simulink model "robot_dynamics_model"  (R2012b)
settings: Solver=ode3  StartTime=0.0  StopTime=inf  FixedStep=0.005  RelTol=1e-3
undefined symbols (not defined in the file or in its folder): x_init
settings Model: ExtModeTrigDuration=5000  Creator=crbonney  LastModifiedBy=crbonney
settings SolverCC: PositivePriorityOrder=on
settings RTWCC: SystemTargetFile=quarc_win64.tlc  TemplateMakefile=quarc_default_tmf  Description=QUARC Win64 Target  ProcessScript=quarc_win64_make_rtw_hook
settings STFCustomTargetCC: TargetPreCompLibLocation=C:\PROGRA~3\QUARC\lib\2012b\win64\release  CodeReplacementLibrary=ANSI_C  GeneratePreprocessorConditionals=Disable all  CombineOutputUpdateFcns=on  GRTInterface=off  SystemTargetFile=quarc_win64.tlc
settings GRTTargetCC: TargetPreCompLibLocation=C:\PROGRA~3\QUARC\lib\2012b\win64\release  ParMdlRefBuildCompliant=off  CompOptLevelCompliant=off  ConcurrentExecutionCompliant=off  MatFileLogging=off  ExtMode=on  ExtModeMexFile=quarc_comm

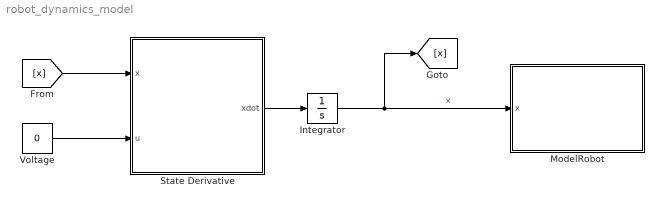
== system robot_dynamics_model ==
  Integrator : Integrator  InitialCondition=x_init
  ModelRobot : MATLAB Function  TreatAsAtomicUnit=on
  State Derivative : MATLAB Function  TreatAsAtomicUnit=on
  Voltage : Constant  Value=0
  wires:
  Integrator/1 -> ModelRobot/1(x), [x]  "x"
  State Derivative/1(xdot) -> Integrator/1
  [x] -> State Derivative/1(x)
  Voltage/1 -> State Derivative/2(u)

== matlab function robot_dynamics_model/ModelRobot ==
  data: x input
function ModelRobot (x)

theta1 = x(1);
theta2 = x(2);

    frame0_links = ...
        [0  0;...  %X
         0  0;...  %Y
         0 -15];   %Z

    frame1_links = ...
        [0  0  0  0 0;... %X
         0  0  6  6 8;... %Y
         0 -1 -1  0 0];   %Z

    frame2_links = ...
        [0   0;... %X
         0  12;... %Y
         0   0];   %Z

    rho = sqrt(8^2+12^2);
    phi_max = atan(12/8);

    f1 = TransformPoints(TRANS0_1(theta1),frame1_links);
    f2 = TransformPoints(TRANS0_1(theta1),TransformPoints(TRANS1_2(theta2),frame2_links));


    plot3(frame0_links(1,:),frame0_links(2,:), frame0_links(3,:),'bs-','LineWidth',3);
    axis([-15 15 -15 15 -15 15]);
    grid on
    hold on
    xlabel('x');
    ylabel('y');
    zlabel('z');
    plot3(f1(1,:),f1(2,:), f1(3,:),'rs-','LineWidth',3);
    plot3(f2(1,:),f2(2,:), f2(3,:),'go-', 'MarkerFaceColor', 'c', 'MarkerSize',5,'LineWidth',3);
    plot3(f2(1,end),f2(2,end), f2(3,end),'go-', 'MarkerFaceColor', 'c', 'MarkerSize',5,'LineWidth',3);
    axis([-15 15 -15 15 -15 15]);
    WorkEnvelope2(rho, phi_max);
    hold off
end

== matlab function robot_dynamics_model/State Derivative ==
  data: x input; u input; xdot output
function xdot = fcn(x, u)

J1 = 0.0012;
m2 = 0.127;
L12 = 0.2;
L2 = 0.3;
Lc2 = L2/2;
beta1 = 0.015;
beta2 = 0.002;
Ra = 2.6;
kt = 0.00768;
kr = 70;
g = 9.81;

theta1 = (J1+m2*L12^2)*Ra/(kr*kt);
theta2 = 1/3*m2*L2^2*Ra/(kr*kt);
theta3 = 1/2*m2*L12*L2*Ra/(kr*kt);
theta4 = m2*Lc2*Ra/(kr*kt);
theta5 = beta1*Ra/(kr*kt)+kr*kt;
theta6 = beta2*Ra/(kr*kt);

q1 = x(1);
q2 = x(2);
q1dot = x(3);
q2dot = x(4);
v = [u; 0];

m =    [...
        (theta1+theta2*sin(q2)^2) (theta3*cos(q2));...
            (theta3*cos(q2)) (theta2);...
];


c =    [...
             (2*theta2*cos(q2)*q2dot) (-theta3*sin(q2)*q2dot);...
         (-theta2*sin(q2)*cos(q2)*q1dot) (0);...
];


f =    [...
         theta5*q1dot;...
         theta6*q2dot;...
];

g =    [...
                  0;...
        -theta4*g*sin(q2);...
];


acceleration = -m\(c*[q1dot;q2dot]+f+g-v);

xdot = [q1dot;q2dot;acceleration];
